simulink model "sim_part1_1"  (R2020a)
settings: Solver=VariableStepAuto  StartTime=0.0  StopTime=10.0  RelTol=1e-3
values from neighbouring files (symbols this model uses):
  gov = 0.5    [a_1.m]    (also in a_2.m; a_loss_function.m; bank_centralbank.m; full_model.m)
  i_cb = 0.03    [a_1.m]    (also in a_2.m = 0.07; a_loss_function.m; full_model.m; part2.m = 0.1)
  i_diff = 0.025    [a_1.m]    (also in a_2.m; a_loss_function.m; bank_and_economy.m = 0.02; full_model.m)
  i_k_p = 0.03    [a_2.m]    (also in part2.m = 0.05; part_1.m = 0.05)
  K_0 = 0.08    [a_1.m]    (also in a_2.m; a_loss_function.m; bank_and_economy.m; bank_centralbank.m)
  K_p = 15    [a_1.m]    (also in a_2.m; a_loss_function.m; bank_and_economy.m = 0.5; bank_centralbank.m)
  lambda = 0.002    [a_1.m]    (also in a_2.m; a_loss_function.m; bank_and_economy.m; bank_centralbank.m)
  lambda_k = 0.005    [a_1.m]    (also in a_2.m; a_loss_function.m; full_model.m; part2.m)
  R = 1    [a_1.m]    (also in a_2.m; a_loss_function.m; bank_and_economy.m; bank_centralbank.m)
  r_k = 0.1    [a_1.m]    (also in a_2.m; a_loss_function.m; bank_and_economy.m; full_model.m)
  rate = 0.1    [a_1.m]    (also in a_2.m; a_loss_function.m; bank_and_economy.m; bank_centralbank.m)
  s_k = 0.25    [a_1.m]    (also in a_2.m; bank_and_economy.m; part2.m = 0.2; part_1.m = 0.2)
  sigma = 0.28    [a_1.m]    (also in a_2.m; a_loss_function.m; bank_and_economy.m; bank_centralbank.m)
  T_f = 0.5    [a_1.m]    (also in a_2.m; a_loss_function.m; bank_and_economy.m; bank_centralbank.m)
  T_g = 1    [a_1.m]    (also in a_2.m; a_loss_function.m; bank_and_economy.m; bank_centralbank.m)
  T_h = 0.1    [a_1.m]    (also in a_2.m; a_loss_function.m; bank_and_economy.m; bank_centralbank.m)
  T_i = 8    [a_1.m]    (also in a_2.m; a_loss_function.m; bank_and_economy.m; bank_centralbank.m)
  T_k = 0.1    [a_1.m]    (also in a_2.m; a_loss_function.m; bank_and_economy.m = 0.25; economy.m = 1)
  tx = 0.3    [a_1.m]    (also in a_2.m; a_loss_function.m; bank_and_economy.m = 0.5; bank_centralbank.m = 0.25)
settings Model: Creator=erlended  LastModifiedBy=erlended

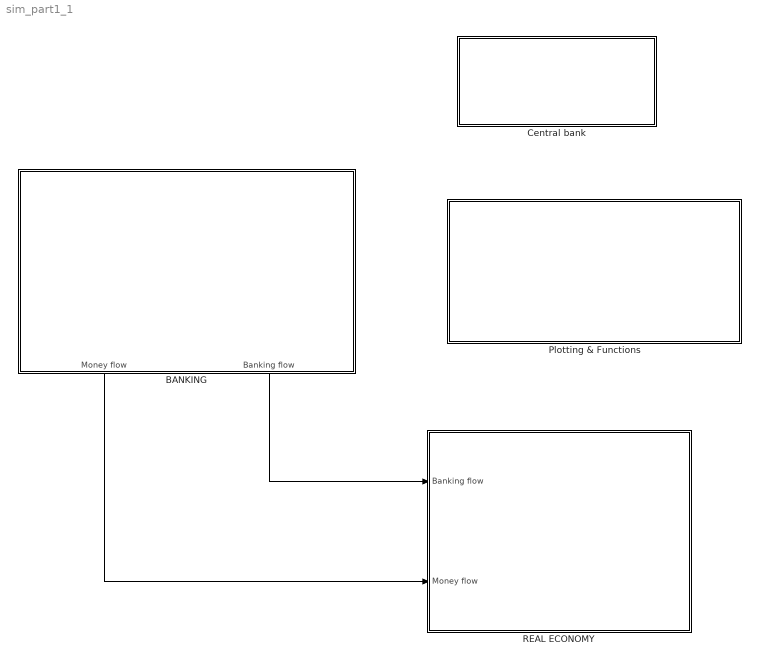
== system sim_part1_1 ==
  BANKING : Subsystem
  "Central bank " : Subsystem
  Plotting & Functions : Subsystem
  REAL ECONOMY : Subsystem
  wires:
  BANKING/2(Banking flow) -> REAL ECONOMY/1(Banking flow)
  BANKING/1(Money flow) -> REAL ECONOMY/2(Money flow)

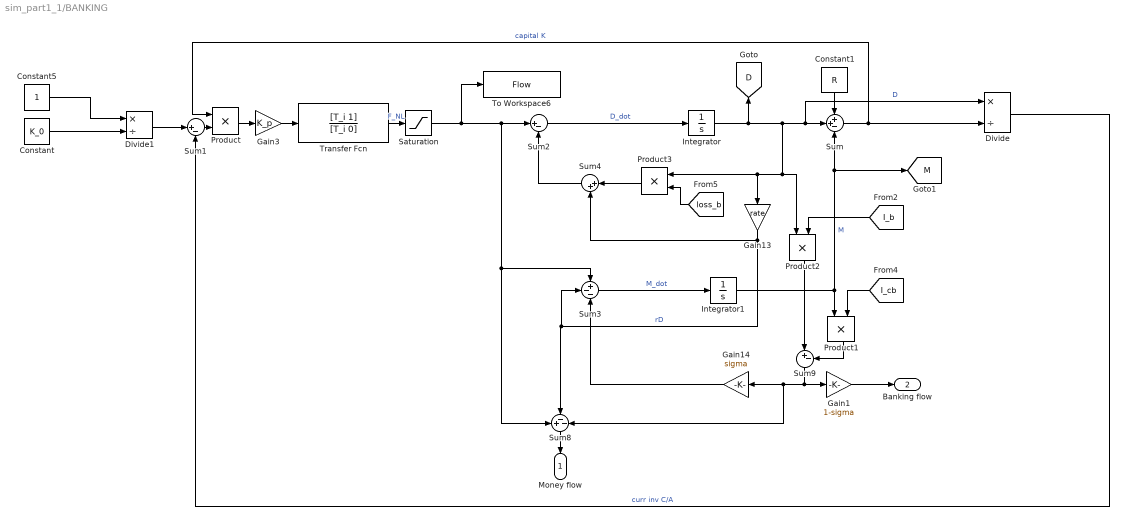
== system sim_part1_1/BANKING ==
  Constant : Constant  Value=K_0
  Constant1 : Constant  Value=R
  Constant5 : Constant
  Divide : Product  Inputs=*/
  Divide1 : Product  Inputs=*/
  Gain1 : Gain  Gain=1-sigma
  Gain13 : Gain  Gain=rate
  Gain14 : Gain  Gain=sigma
  Gain3 : Gain  Gain=K_p
  Integrator : Integrator
  Integrator1 : Integrator
  Product{,1..3} (4 alike) : Product
  Saturation : Saturate  UpperLimit=1000  LowerLimit=0
  Sum : Sum  Inputs=++-
  Sum1 : Sum  Inputs=|+-
  Sum2 : Sum  Inputs=|+-
  Sum3 : Sum  Inputs=+--
  Sum4 : Sum  Inputs=|++
  Sum8 : Sum  Inputs=+--
  Sum9 : Sum  Inputs=|+-
  To Workspace6 : ToWorkspace  VariableName=Flow  SaveFormat=Timeseries  SampleTime=-1
  Transfer Fcn : TransferFcn  Numerator=[T_i 1]  Denominator=[T_i 0]
  Money flow : Outport
  Banking flow : Outport  Port=2
  tag scope: D=global, M=global
  wires:
  Product/1 -> Gain3/1
  Integrator/1 -> Sum/2, Divide/1, Product3/1, Gain13/1, Product2/1, [D]  "D"
  Sum8/1 -> Money flow/1
  Integrator1/1 -> [M], Sum/3, Product1/1  "M"
  Saturation/1 -> Sum2/1, Sum3/1, Sum8/1, To Workspace6/1
  Transfer Fcn/1 -> Saturation/1  "F_NL"
  Sum/1 -> Product/1, Divide/2  "capital K"
  Sum4/1 -> Sum2/2
  Gain13/1 -> Sum4/2, Sum8/2, Sum3/2  "rD"
  Sum9/1 -> Gain1/1, Sum8/3, Gain14/1
  Sum2/1 -> Integrator/1  "D_dot"
  Gain3/1 -> Transfer Fcn/1
  Constant1/1 -> Sum/1
  Divide/1 -> Sum1/2  "curr inv C/A"
  Sum1/1 -> Product/2
  Sum3/1 -> Integrator1/1  "M_dot"
  Product2/1 -> Sum9/1
  Product1/1 -> Sum9/2
  Constant5/1 -> Divide1/1
  Divide1/1 -> Sum1/1
  Gain14/1 -> Sum3/3
  Gain1/1 -> Banking flow/1
  Constant/1 -> Divide1/2
  [I_b] -> Product2/2
  [I_cb] -> Product1/2
  Product3/1 -> Sum4/1
  [loss_b] -> Product3/2

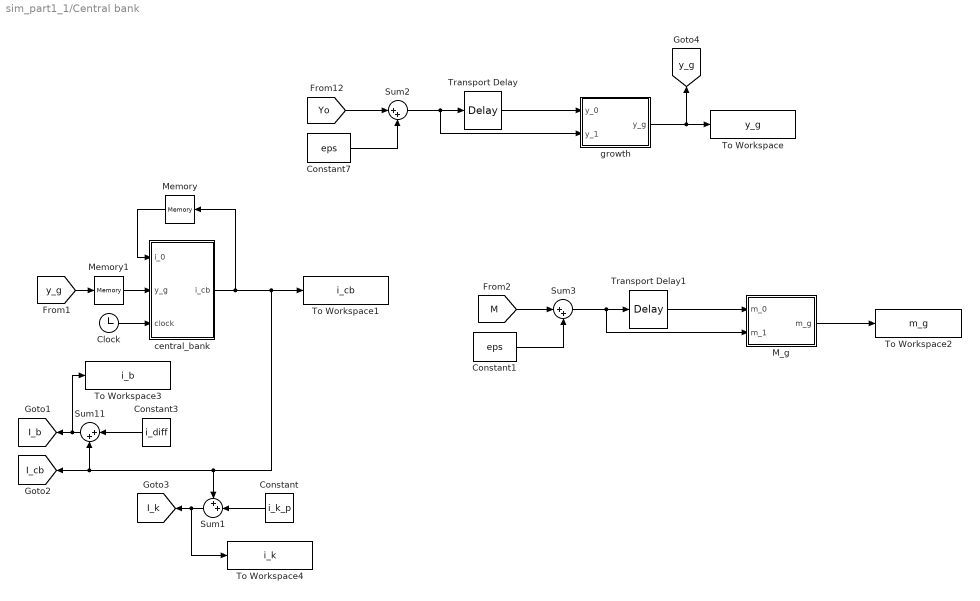
== system sim_part1_1/Central bank  ==
  Clock : Clock
  Constant : Constant  Value=i_k_p
  Constant1 : Constant  Value=eps
  Constant3 : Constant  Value=i_diff
  Constant7 : Constant  Value=eps
  M_g : MATLAB Function  TreatAsAtomicUnit=on
  Memory : Memory  InitialCondition=i_cb
  Memory1 : Memory
  Sum1 : Sum  Inputs=++|
  Sum11 : Sum  Inputs=|++
  Sum2 : Sum  Inputs=|++
  Sum3 : Sum  Inputs=|++
  To Workspace : ToWorkspace  VariableName=y_g  SaveFormat=Timeseries  SampleTime=-1
  To Workspace1 : ToWorkspace  VariableName=i_cb  SaveFormat=Timeseries  SampleTime=-1
  To Workspace2 : ToWorkspace  VariableName=m_g  SaveFormat=Timeseries  SampleTime=-1
  To Workspace3 : ToWorkspace  VariableName=i_b  SaveFormat=Timeseries  SampleTime=-1
  To Workspace4 : ToWorkspace  VariableName=i_k  SaveFormat=Timeseries  SampleTime=-1
  Transport Delay : TransportDelay
  Transport Delay1 : TransportDelay
  central_bank : MATLAB Function  TreatAsAtomicUnit=on
  growth : MATLAB Function  TreatAsAtomicUnit=on
  tag scope: I_b=global, I_cb=global, I_k=global, y_g=global
  wires:
  Constant/1 -> Sum1/2
  Sum1/1 -> To Workspace4/1, [I_k]
  Constant3/1 -> Sum11/1
  Sum11/1 -> To Workspace3/1, [I_b]
  Constant7/1 -> Sum2/2
  [Yo] -> Sum2/1
  Sum2/1 -> Transport Delay/1, growth/2(y_1)
  growth/1(y_g) -> [y_g], To Workspace/1
  Transport Delay/1 -> growth/1(y_0)
  [y_g] -> Memory1/1
  Memory/1 -> central_bank/1(i_0)
  Clock/1 -> central_bank/3(clock)
  Memory1/1 -> central_bank/2(y_g)
  M_g/1(m_g) -> To Workspace2/1
  Sum3/1 -> Transport Delay1/1, M_g/2(m_1)
  Constant1/1 -> Sum3/2
  Transport Delay1/1 -> M_g/1(m_0)
  [M] -> Sum3/1
  central_bank/1(i_cb) -> Memory/1, To Workspace1/1, [I_cb], Sum11/2, Sum1/1

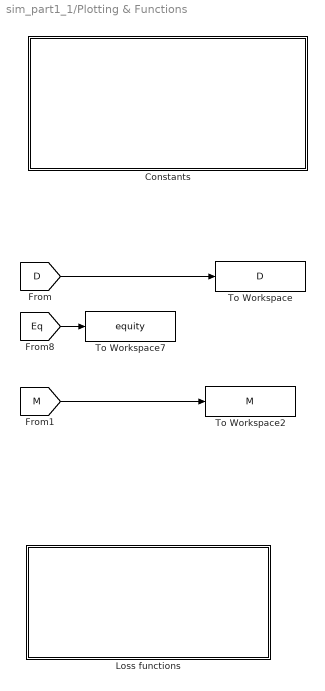
== system sim_part1_1/Plotting & Functions ==
  Constants : Subsystem
  Loss functions : Subsystem
  To Workspace : ToWorkspace  VariableName=D  SaveFormat=Timeseries  SampleTime=-1
  To Workspace2 : ToWorkspace  VariableName=M  SaveFormat=Timeseries  SampleTime=-1
  To Workspace7 : ToWorkspace  VariableName=equity  SaveFormat=Timeseries  SampleTime=-1
  wires:
  [D] -> To Workspace/1
  [Eq] -> To Workspace7/1
  [M] -> To Workspace2/1

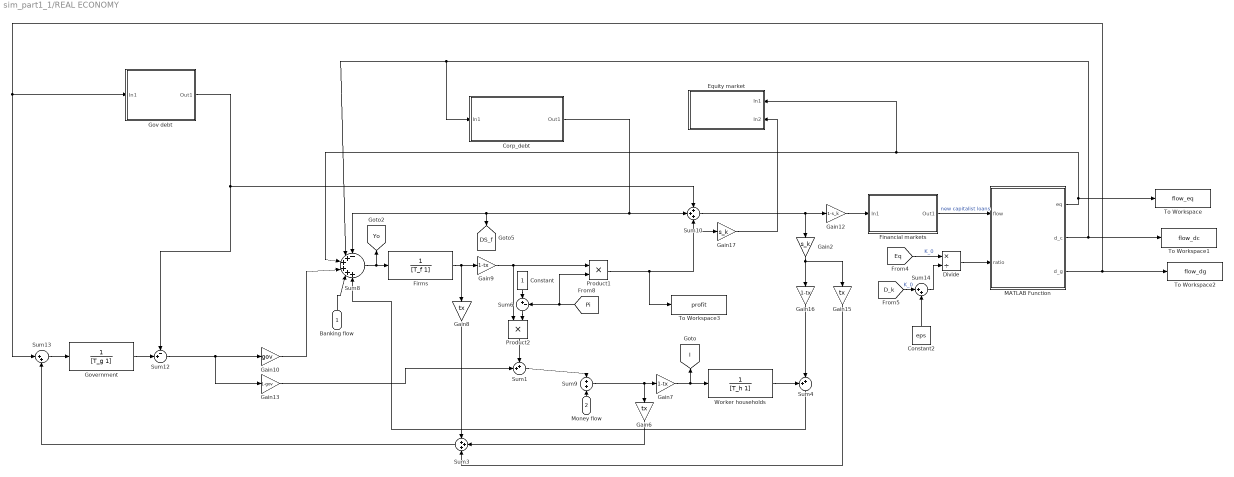
== system sim_part1_1/REAL ECONOMY ==
  Banking flow : Inport
  Money flow : Inport  Port=2
  Constant : Constant
  Constant2 : Constant  Value=eps
  Corp_debt : Subsystem
  Divide : Product  Inputs=*/
  Equity market : Subsystem
  Financial markets : Subsystem
  Firms : TransferFcn  Denominator=[T_f 1]
  Gain10 : Gain  Gain=gov
  Gain12 : Gain  Gain=1-s_k
  Gain13 : Gain  Gain=1-gov
  Gain15 : Gain  Gain=tx
  Gain16 : Gain  Gain=1-tx
  Gain17 : Gain  Gain=s_k
  Gain2 : Gain  Gain=s_k
  Gain6 : Gain  Gain=tx
  Gain7 : Gain  Gain=1-tx
  Gain8 : Gain  Gain=tx
  Gain9 : Gain  Gain=1-tx
  Gov debt : Subsystem
  Government : TransferFcn  Denominator=[T_g 1]
  MATLAB Function : MATLAB Function  TreatAsAtomicUnit=on
  Product1 : Product
  Product2 : Product
  Sum1 : Sum  Inputs=++|
  Sum10 : Sum  Inputs=+++
  Sum12 : Sum  Inputs=-+|
  Sum13 : Sum  Inputs=|++
  Sum14 : Sum  Inputs=|++
  Sum3 : Sum  Inputs=+++
  Sum4 : Sum  Inputs=++|
  Sum6 : Sum  Inputs=|+-
  Sum8 : Sum  Inputs=-+++++
  Sum9 : Sum
  To Workspace : ToWorkspace  VariableName=flow_eq  SaveFormat=Timeseries  SampleTime=-1
  To Workspace1 : ToWorkspace  VariableName=flow_dc  SaveFormat=Timeseries  SampleTime=-1
  To Workspace2 : ToWorkspace  VariableName=flow_dg  SaveFormat=Timeseries  SampleTime=-1
  To Workspace3 : ToWorkspace  VariableName=profit  SaveFormat=Timeseries  SampleTime=-1
  Worker households : TransferFcn  Denominator=[T_h 1]
  tag scope: DS_f=global, I=global, Yo=global
  wires:
  Sum8/1 -> [Yo], Firms/1
  Product1/1 -> To Workspace3/1, Sum10/3, Gain17/1
  Sum9/1 -> Gain7/1, Gain6/1
  Firms/1 -> Gain8/1, Gain9/1
  Gain7/1 -> [I], Worker households/1
  Gain8/1 -> Sum3/1
  Gain6/1 -> Sum3/2
  Product2/1 -> Sum1/1
  Sum1/1 -> Sum9/1
  Gain13/1 -> Sum1/2
  Banking flow/1 -> Sum8/5
  Gain10/1 -> Sum8/4
  Financial markets/1(Out1) -> MATLAB Function/1(flow)  "new capitalist loans"
  Worker households/1 -> Sum4/1
  Sum4/1 -> Sum8/6
  Sum10/1 -> Gain12/1, Gain2/1
  Gain2/1 -> Gain15/1, Gain16/1
  Gain15/1 -> Sum3/3
  Gain16/1 -> Sum4/2
  [Pi] -> Sum6/2, Product1/2
  Gain9/1 -> Product2/1, Product1/1
  Sum6/1 -> Product2/2
  Constant/1 -> Sum6/1
  Government/1 -> Sum12/2
  Sum12/1 -> Gain13/1, Gain10/1
  Sum3/1 -> Sum13/2
  Sum13/1 -> Government/1
  [Eq] -> Divide/1  "K_0"
  Divide/1 -> MATLAB Function/2(ratio)
  [D_k] -> Sum14/1  "K_0"
  Sum14/1 -> Divide/2
  Constant2/1 -> Sum14/2
  Money flow/1 -> Sum9/2
  Corp_debt/1(Out1) -> Sum10/2, [DS_f], Sum8/1
  Gov debt/1(Out1) -> Sum12/1, Sum10/1
  Gain17/1 -> Equity market/2(In2)
  Gain12/1 -> Financial markets/1(In1)
  MATLAB Function/2(d_c) -> To Workspace1/1, Corp_debt/1(In1), Sum8/2
  MATLAB Function/3(d_g) -> To Workspace2/1, Gov debt/1(In1), Sum13/1
  MATLAB Function/1(eq) -> To Workspace/1, Equity market/1(In1), Sum8/3

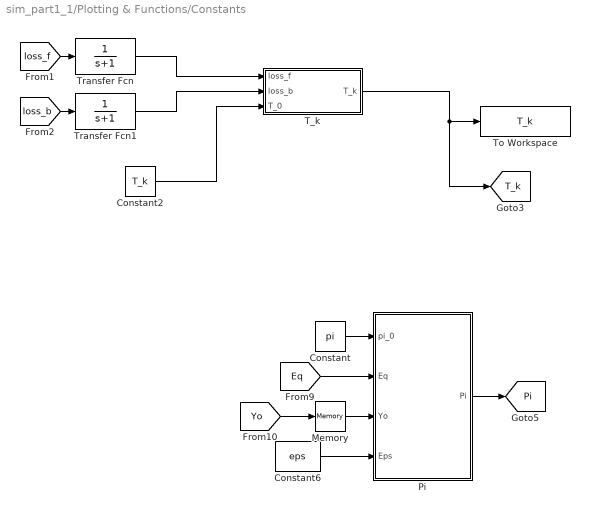
== system sim_part1_1/Plotting & Functions/Constants ==
  Constant : Constant  Value=pi
  Constant2 : Constant  Value=T_k
  Constant6 : Constant  Value=eps
  Memory : Memory
  Pi : MATLAB Function  TreatAsAtomicUnit=on
  T_k : MATLAB Function  TreatAsAtomicUnit=on
  To Workspace : ToWorkspace  VariableName=T_k  SaveFormat=Timeseries  SampleTime=-1
  Transfer Fcn : TransferFcn  Denominator=[1 1]
  Transfer Fcn1 : TransferFcn  Denominator=[1 1]
  tag scope: Pi=global, T_k=global
  wires:
  Pi/1(Pi) -> [Pi]
  T_k/1(T_k) -> [T_k], To Workspace/1
  [Eq] -> Pi/2(Eq)
  Memory/1 -> Pi/3(Yo)
  Constant/1 -> Pi/1(pi_0)
  [Yo] -> Memory/1
  Constant2/1 -> T_k/3(T_0)
  Constant6/1 -> Pi/4(Eps)
  Transfer Fcn/1 -> T_k/1(loss_f)
  [loss_f] -> Transfer Fcn/1
  [loss_b] -> Transfer Fcn1/1
  Transfer Fcn1/1 -> T_k/2(loss_b)

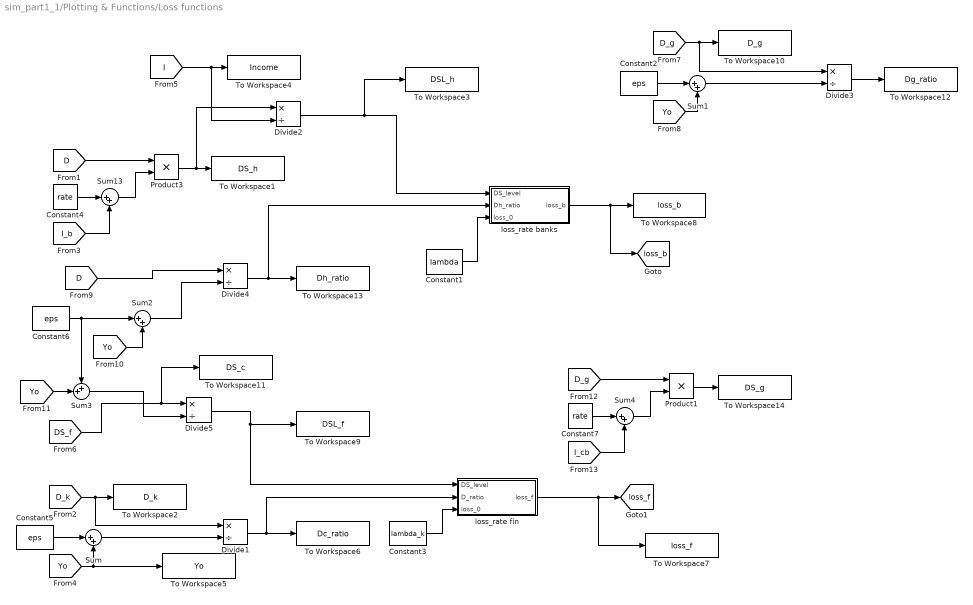
== system sim_part1_1/Plotting & Functions/Loss functions ==
  Constant1 : Constant  Value=lambda
  Constant2 : Constant  Value=eps
  Constant3 : Constant  Value=lambda_k
  Constant4 : Constant  Value=rate
  Constant5 : Constant  Value=eps
  Constant6 : Constant  Value=eps
  Constant7 : Constant  Value=rate
  Divide{1..5} (5 alike) : Product  Inputs=*/
  Product1 : Product
  Product3 : Product
  Sum{,1..2,4,13} (5 alike) : Sum  Inputs=|++
  Sum3 : Sum  Inputs=++|
  To Workspace1 : ToWorkspace  VariableName=DS_h  SaveFormat=Timeseries  SampleTime=-1
  To Workspace10 : ToWorkspace  VariableName=D_g  SaveFormat=Timeseries  SampleTime=-1
  To Workspace11 : ToWorkspace  VariableName=DS_c  SaveFormat=Timeseries  SampleTime=-1
  To Workspace12 : ToWorkspace  VariableName=Dg_ratio  SaveFormat=Timeseries  SampleTime=-1
  To Workspace13 : ToWorkspace  VariableName=Dh_ratio  SaveFormat=Timeseries  SampleTime=-1
  To Workspace14 : ToWorkspace  VariableName=DS_g  SaveFormat=Timeseries  SampleTime=-1
  To Workspace2 : ToWorkspace  VariableName=D_k  SaveFormat=Timeseries  SampleTime=-1
  To Workspace3 : ToWorkspace  VariableName=DSL_h  SaveFormat=Timeseries  SampleTime=-1
  To Workspace4 : ToWorkspace  VariableName=Income  SaveFormat=Timeseries  SampleTime=-1
  To Workspace5 : ToWorkspace  VariableName=Yo  SaveFormat=Timeseries  SampleTime=-1
  To Workspace6 : ToWorkspace  VariableName=Dc_ratio  SaveFormat=Timeseries  SampleTime=-1
  To Workspace7 : ToWorkspace  VariableName=loss_f  SaveFormat=Timeseries  SampleTime=-1
  To Workspace8 : ToWorkspace  VariableName=loss_b  SaveFormat=Timeseries  SampleTime=-1
  To Workspace9 : ToWorkspace  VariableName=DSL_f  SaveFormat=Timeseries  SampleTime=-1
  loss_rate banks : MATLAB Function  TreatAsAtomicUnit=on
  loss_rate fin : MATLAB Function  TreatAsAtomicUnit=on
  tag scope: loss_b=global, loss_f=global
  wires:
  Sum/1 -> Divide1/2
  Constant1/1 -> loss_rate banks/3(loss_0)
  Constant5/1 -> Sum/1
  [D_k] -> To Workspace2/1, Divide1/1
  Constant4/1 -> Sum13/1
  Product3/1 -> Divide2/1, To Workspace1/1
  [D] -> Product3/1
  [I_b] -> Sum13/2
  [I] -> Divide2/2, To Workspace4/1
  loss_rate banks/1(loss_b) -> [loss_b], To Workspace8/1
  Sum13/1 -> Product3/2
  [Yo] -> Sum/2, To Workspace5/1
  Divide1/1 -> loss_rate fin/2(D_ratio), To Workspace6/1
  loss_rate fin/1(loss_f) -> To Workspace7/1, [loss_f]
  Constant3/1 -> loss_rate fin/3(loss_0)
  [Yo] -> Sum1/2
  Constant2/1 -> Sum1/1
  Sum1/1 -> Divide3/2
  [D_g] -> To Workspace10/1, Divide3/1
  Divide3/1 -> To Workspace12/1
  Constant6/1 -> Sum3/1, Sum2/1
  Sum2/1 -> Divide4/2
  [D] -> Divide4/1
  Divide4/1 -> loss_rate banks/2(Dh_ratio), To Workspace13/1
  [Yo] -> Sum2/2
  Divide2/1 -> To Workspace3/1, loss_rate banks/1(DS_level)
  [DS_f] -> To Workspace11/1, Divide5/1
  Divide5/1 -> To Workspace9/1, loss_rate fin/1(DS_level)
  [Yo] -> Sum3/2
  Sum3/1 -> Divide5/2
  Sum4/1 -> Product1/2
  [I_cb] -> Sum4/2
  Constant7/1 -> Sum4/1
  [D_g] -> Product1/1
  Product1/1 -> To Workspace14/1

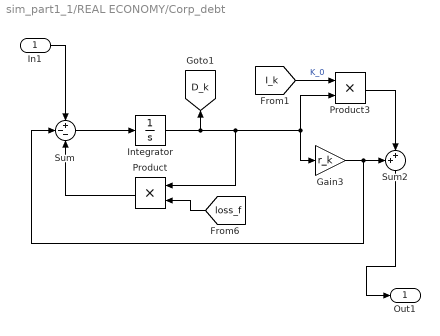
== system sim_part1_1/REAL ECONOMY/Corp_debt ==
  In1 : Inport
  Gain3 : Gain  Gain=r_k
  Integrator : Integrator
  Product : Product
  Product3 : Product
  Sum : Sum  Inputs=+--
  Sum2 : Sum  Inputs=++|
  Out1 : Outport
  tag scope: D_k=global
  wires:
  Product/1 -> Sum/3
  In1/1 -> Sum/1
  Sum2/1 -> Out1/1
  [loss_f] -> Product/2
  [I_k] -> Product3/1  "K_0"
  Sum/1 -> Integrator/1
  Integrator/1 -> [D_k], Product/1, Product3/2, Gain3/1
  Product3/1 -> Sum2/2
  Gain3/1 -> Sum/2, Sum2/1

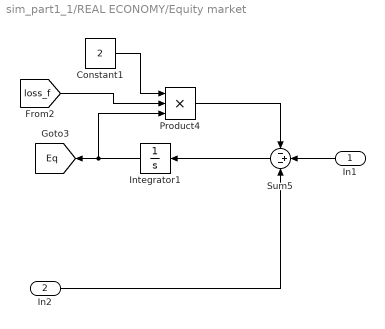
== system sim_part1_1/REAL ECONOMY/Equity market ==
  In1 : Inport
  In2 : Inport  Port=2
  Constant1 : Constant  Value=2
  Integrator1 : Integrator
  Product4 : Product  Inputs=3
  Sum5 : Sum  Inputs=-+-
  tag scope: Eq=global
  wires:
  Sum5/1 -> Integrator1/1
  Constant1/1 -> Product4/1
  In2/1 -> Sum5/3
  Product4/1 -> Sum5/1
  In1/1 -> Sum5/2
  Integrator1/1 -> Product4/3, [Eq]
  [loss_f] -> Product4/2

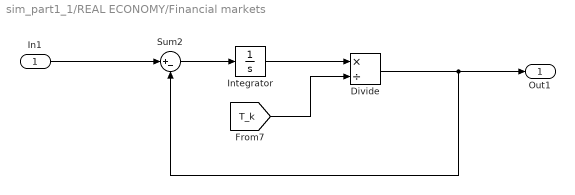
== system sim_part1_1/REAL ECONOMY/Financial markets ==
  In1 : Inport
  Divide : Product  Inputs=*/
  Integrator : Integrator
  Sum2 : Sum  Inputs=|+-
  Out1 : Outport
  wires:
  In1/1 -> Sum2/1
  Sum2/1 -> Integrator/1
  Divide/1 -> Out1/1, Sum2/2
  Integrator/1 -> Divide/1
  [T_k] -> Divide/2

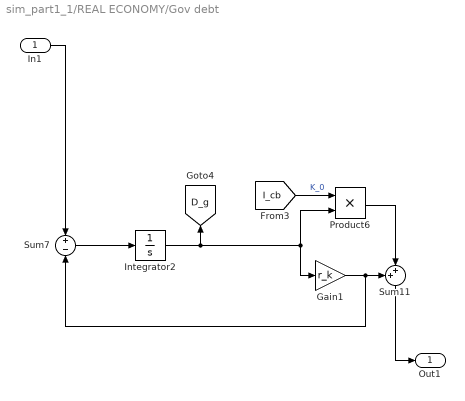
== system sim_part1_1/REAL ECONOMY/Gov debt ==
  In1 : Inport
  Gain1 : Gain  Gain=r_k
  Integrator2 : Integrator
  Product6 : Product
  Sum11 : Sum  Inputs=++|
  Sum7 : Sum  Inputs=+-
  Out1 : Outport
  tag scope: D_g=global
  wires:
  Integrator2/1 -> [D_g], Product6/2, Gain1/1
  Sum7/1 -> Integrator2/1
  In1/1 -> Sum7/1
  [I_cb] -> Product6/1  "K_0"
  Gain1/1 -> Sum7/2, Sum11/1
  Product6/1 -> Sum11/2
  Sum11/1 -> Out1/1

== matlab function sim_part1_1/Plotting & Functions/Loss functions/loss_rate banks ==
  data: DS_level input; Dh_ratio input; loss_b output; loss_0 input
function loss_b = fcn(DS_level, Dh_ratio,loss_0)

loss_b = 0.0025*(Dh_ratio/1.6)^6+0.05*DS_level^6+loss_0;

%if loss_b > 0.01
%    loss_b = 0.01;
%end

== matlab function sim_part1_1/REAL ECONOMY/MATLAB Function ==
  data: flow input; eq output; d_c output; d_g output; ratio input
function [eq,d_c,d_g]= fcn(flow, ratio)
d_g = flow*0.2;

if ratio > 1
    eq = flow*(0.5 - 0.15*ratio);
    d_c = flow*(0.3 + 0.15*ratio);
else
    eq = flow*(0.5 + 0.15*ratio);
    d_c = flow*(0.3 - 0.15*ratio);
end

== matlab function sim_part1_1/Plotting & Functions/Loss functions/loss_rate fin ==
  data: DS_level input; D_ratio input; loss_f output; loss_0 input
function loss_f = fcn(DS_level, D_ratio,loss_0)

%loss_f = 0.0015*(D_ratio)^4+loss_0;

loss_f = 0.0015*(D_ratio)^4+(1.5*DS_level)^4+loss_0;

%if loss_f > 0.05
%    loss_f = 0.05;
%end

== matlab function sim_part1_1/Plotting & Functions/Constants/T_k ==
  data: loss_f input; loss_b input; T_k output; T_0 input
function T_k = fcn(loss_f, loss_b, T_0)

%T_k = 0.55*(0.998+400*my)*T_0;
%T_k = 0.03*(ratio)^2+2*my+T_0;
T_k = 15*loss_f+60*loss_b+T_0;

== matlab function sim_part1_1/Plotting & Functions/Constants/Pi ==
  data: pi_0 input; Pi output; Eq input; Yo input; Eps input
function Pi = fcn(pi_0, Eq, Yo, Eps)

Pi = 0.05*Eq/(Yo+Eps)+pi_0;
if Pi > 0.6
    Pi = 0.6; 
end

== matlab function sim_part1_1/Central bank /growth ==
  data: y_0 input; y_g output; y_1 input
function y_g = fcn(y_0, y_1)

y_g = (y_1-y_0)/y_0;

== matlab function sim_part1_1/Central bank /central_bank ==
  data: i_0 input; y_g input; i_cb output; clock input
function i_cb = fcn(i_0, y_g, clock)

i_cb = i_0;

if y_g < 0.01 && clock > 5
    i_cb = i_0 - 0.005;
elseif y_g > 0.06 && clock > 5
   i_cb = i_0 + 0.0025;
end

if i_cb <= 0
    i_cb = 0;
end

== matlab function sim_part1_1/Central bank /M_g ==
  data: m_0 input; m_g output; m_1 input
function m_g = fcn(m_0, m_1)

m_g = (m_1-m_0)/m_0;
